simulink model "a1be3d"  (R2021a)
settings: Solver=VariableStepAuto  StartTime=0.0  StopTime=10.0  RelTol=1e-3
values from neighbouring files (symbols this model uses):
  b = 0.36    [a1be3.mat]
  c1 = 0.86    [a1be3.mat]
  c2 = 33.82    [a1be3.mat]
  c3 = 0.36    [a1be3.mat]
  g = 9.81    [a1be3.mat]
  JR = 0.8    [a1be3.mat]
  lambda_max = 0.1298    [a1be3.mat]
  m = 1300    [a1be3.mat]    (also in a1be3c.m = find(fc == max(fc)))
  rR = 0.3    [a1be3.mat]
libraries: pid_lib x1
settings Model: Creator=Ans Shahzad  LastModifiedBy=Ans Shahzad

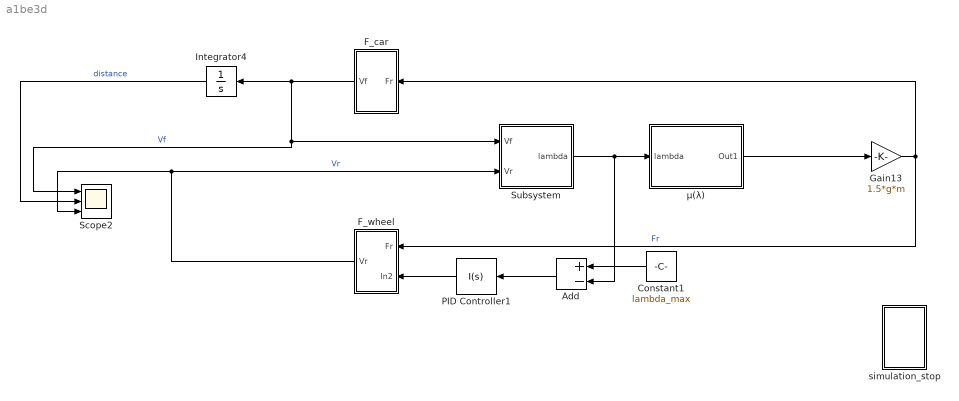
== system a1be3d ==
  Add : Sum  Inputs=+-
  Constant1 : Constant  Value=lambda_max
  F_car : Subsystem
  F_wheel : Subsystem
  Gain13 : Gain  Gain=1.5*g*m
  Integrator4 : Integrator
  PID Controller1 : pid_lib/PID Controller  Controller=I  Form=Parallel  TimeDomain=Continuous-time  UseExternalTs=off  SampleTime=-1  IntegratorMethod=Forward Euler  FilterMethod=Forward Euler  ControllerParametersSource=internal  P=1  I=100000  D=0  UseFilter=on  N=100  TunerSelectOption=Transfer Function Based (PID Tuner App)  ZeroCross=off  InitialConditionSource=internal  InitialConditionForIntegrator=0  InitialConditionForFilter=0  DifferentiatorICPrevScaledInput=0  ExternalReset=none  TrackingMode=off  Kt=1  LimitOutput=off  SatLimitsSource=external  UpperSaturationLimit=inf  LowerSaturationLimit=0  LinearizeAsGain=on  AntiWindupMode=none  Kb=1  POutMin=[]  POutMax=[]  IOutMin=[]  IOutMax=[]  DOutMin=[]  DOutMax=[]  NOutMin=[]  NOutMax=[]  SumOutMin=[]  SumOutMax=[]  SaturationOutMin=[]  SaturationOutMax=[]  PParamMin=[]  PParamMax=[]  IParamMin=[]  IParamMax=[]  DParamMin=[]  DParamMax=[]  NParamMin=[]  NParamMax=[]  KbParamMin=[]  KbParamMax=[]  KtParamMin=[]  KtParamMax=[]  KbOutMin=[]  KbOutMax=[]  KtOutMin=[]  KtOutMax=[]  IntegratorOutMin=[]  IntegratorOutMax=[]  FilterOutMin=[]  FilterOutMax=[]  SumI1OutMin=[]  SumI1OutMax=[]  SumI2OutMin=[]  SumI2OutMax=[]  SumI3OutMin=[]  SumI3OutMax=[]  SumI4OutMin=[]  SumI4OutMax=[]  SumDOutMin=[]  SumDOutMax=[]  DifferentiatorOutMin=[]  DifferentiatorOutMax=[]  FilterDiffOutCoefMin=[]  FilterDiffOutCoefMax=[]  ReciprocalOutMin=[]  ReciprocalOutMax=[]  SumDenOutMin=[]  SumDenOutMax=[]  SumNumOutMin=[]  SumNumOutMax=[]  DivideOutMin=[]  DivideOutMax=[]  UdiffTsProdOutMin=[]  UdiffTsProdOutMax=[]  NTsProdOutMin=[]  NTsProdOutMax=[]  UintegralTsProdOutMin=[]  UintegralTsProdOutMax=[]  UngainTsProdOutMin=[]  UngainTsProdOutMax=[]  IntegratorContinuousStateAttributes=''  IntegratorStateMustResolveToSignalObject=off  IntegratorRTWStateStorageClass=Auto  FilterContinuousStateAttributes=''  FilterStateMustResolveToSignalObject=off  FilterRTWStateStorageClass=Auto  ParallelPVariant=Disabled  IdealPVariant=Disabled  IVariant=InternalParameters  DVariant=Disabled  IntegratorVariant=Continuous  SatVariant=Disabled  AWVariant=Passthrough  PCopyVariant=Disabled  TRVariant=Disabled  FdbkBlocksVariant=Forward  IdealPFdbkVariant=Disabled  SatFdbkVariant=Disabled  DerivativeFilterVariant=Disabled  NVariant=Disabled  NCopyVariant=Disabled_SignalSpec  FilterICVariant=Disabled  IntegratorICVariant=InternalICs  ExternalResetVariant=Disabled  TRSumVariant=Passthrough  SumFdbkVariant=Disabled  SumVariant=Passthrough_I  TsampFilterVariant=InternalTs  TsampNgainVariant=Passthrough  TsampIntegralVariant=Passthrough  ExternalSaturationOutDataTypeStr=Inherit: Same as second input
  Scope2 : Scope  NumInputPorts=3
  Subsystem : Subsystem
  simulation_stop : Subsystem
  "µ(λ) " : Subsystem
  wires:
  Gain13/1 -> F_wheel/1(Fr), F_car/1(Fr)  "Fr"
  Integrator4/1 -> Scope2/2  "distance"
  Constant1/1 -> Add/1
  Add/1 -> PID Controller1/1
  "µ(λ) "/1(Out1) -> Gain13/1
  Subsystem/1(lambda) -> "µ(λ) "/1(lambda), Add/2
  F_wheel/1(Vr) -> Scope2/3, Subsystem/2(Vr)  "Vr"
  PID Controller1/1 -> F_wheel/2(In2)
  F_car/1(Vf) -> Subsystem/1(Vf), Scope2/1, Integrator4/1  "Vf"

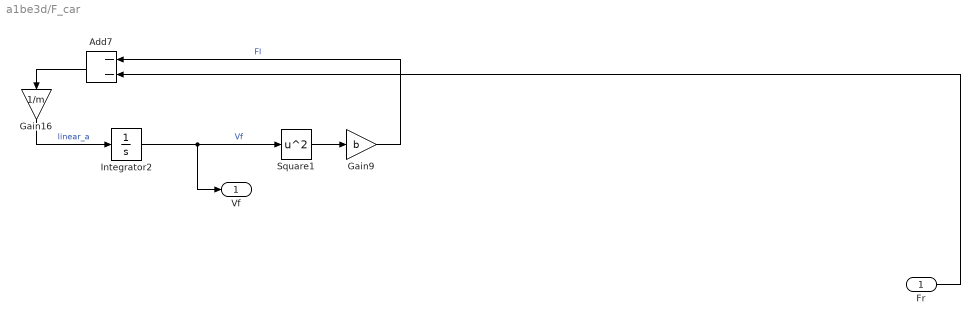
== system a1be3d/F_car ==
  Fr : Inport
  Add7 : Sum  Inputs=--
  Gain16 : Gain  Gain=1/m
  Gain9 : Gain  Gain=b
  Integrator2 : Integrator  InitialCondition=30  LimitOutput=on  UpperSaturationLimit=1000  LowerSaturationLimit=0  ZeroCross=off
  Square1 : Math  Operator=square  SaturateOnIntegerOverflow=on
  Vf : Outport
  wires:
  Square1/1 -> Gain9/1
  Gain16/1 -> Integrator2/1  "linear_a"
  Integrator2/1 -> Vf/1, Square1/1  "Vf"
  Add7/1 -> Gain16/1
  Gain9/1 -> Add7/1  "Fl"
  Fr/1 -> Add7/2

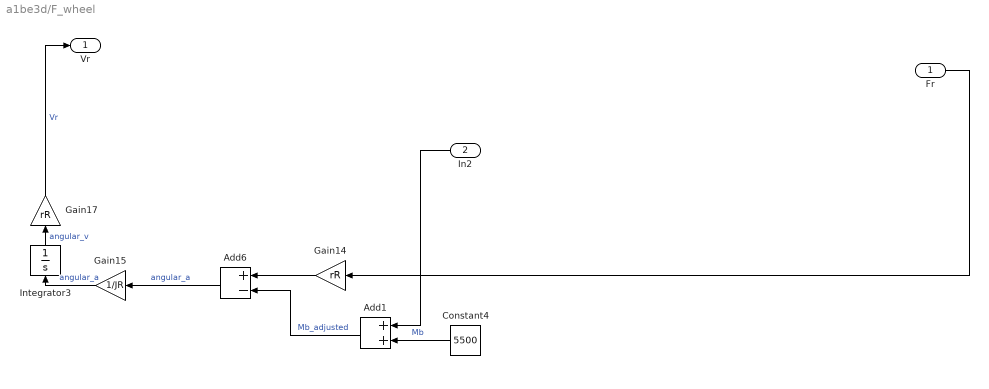
== system a1be3d/F_wheel ==
  Fr : Inport
  In2 : Inport  Port=2
  Add1 : Sum
  Add6 : Sum  Inputs=+-
  Constant4 : Constant  Value=5500
  Gain14 : Gain  Gain=rR
  Gain15 : Gain  Gain=1/JR
  Gain17 : Gain  Gain=rR
  Integrator3 : Integrator  InitialCondition=100  LimitOutput=on  UpperSaturationLimit=1000  LowerSaturationLimit=0
  Vr : Outport
  wires:
  Gain17/1 -> Vr/1  "Vr"
  Gain14/1 -> Add6/1
  Add6/1 -> Gain15/1  "angular_a"
  Gain15/1 -> Integrator3/1  "angular_a"
  Integrator3/1 -> Gain17/1  "angular_v"
  Add1/1 -> Add6/2  "Mb_adjusted"
  Constant4/1 -> Add1/2  "Mb"
  Fr/1 -> Gain14/1
  In2/1 -> Add1/1

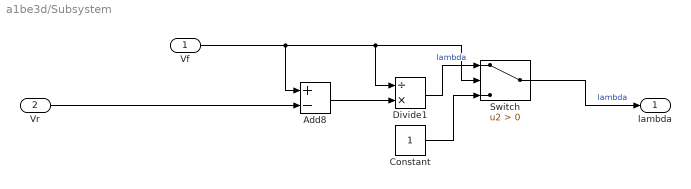
== system a1be3d/Subsystem ==
  Vf : Inport
  Vr : Inport  Port=2
  Add8 : Sum  Inputs=+-
  Constant : Constant
  Divide1 : Product  Inputs=/*
  Switch : Switch  Criteria=u2 > Threshold
  lambda : Outport
  wires:
  Add8/1 -> Divide1/2
  Vf/1 -> Divide1/1, Switch/2, Add8/1
  Switch/1 -> lambda/1  "lambda"
  Divide1/1 -> Switch/1  "lambda"
  Constant/1 -> Switch/3
  Vr/1 -> Add8/2

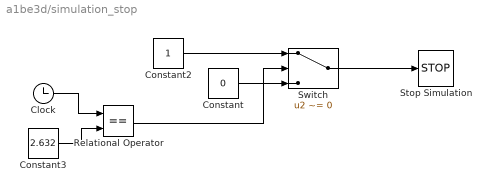
== system a1be3d/simulation_stop ==
  Clock : Clock
  Constant : Constant  Value=0
  Constant2 : Constant
  Constant3 : Constant  Value=2.632
  Relational Operator : RelationalOperator  Operator===  OutDataTypeStr=boolean  RndMeth=Simplest
  Stop Simulation : Stop
  Switch : Switch  Criteria=u2 ~= 0  RndMeth=Nearest
  wires:
  Constant2/1 -> Switch/1
  Switch/1 -> Stop Simulation/1
  Constant3/1 -> Relational Operator/2
  Relational Operator/1 -> Switch/2
  Constant/1 -> Switch/3
  Clock/1 -> Relational Operator/1

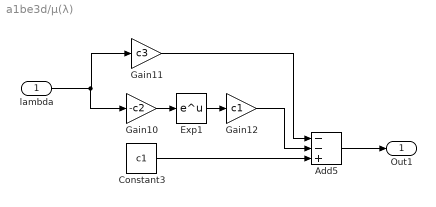
== system a1be3d/µ(λ)  ==
  lambda : Inport
  Add5 : Sum  Inputs=--+
  Constant3 : Constant  Value=c1
  Exp1 : Math  SaturateOnIntegerOverflow=on
  Gain10 : Gain  Gain=-c2
  Gain11 : Gain  Gain=c3
  Gain12 : Gain  Gain=c1
  Out1 : Outport
  wires:
  Gain12/1 -> Add5/2
  lambda/1 -> Gain10/1, Gain11/1
  Gain11/1 -> Add5/1
  Gain10/1 -> Exp1/1
  Exp1/1 -> Gain12/1
  Constant3/1 -> Add5/3
  Add5/1 -> Out1/1
